simulink model "PurePursuitAlgorithm"  (R2022a)
settings: Solver=ode23t  StartTime=0.0  StopTime=inf  RelTol=1e-3
InitFcn:
  | RPInit
undefined symbols (not defined in the file or in its folder): xRef1, yRef1
libraries: RoboticsPlayground x2
settings Model: Creator=berke  LastModifiedBy=berke
settings DebuggingCC: UnconnectedInputMsg=warning  UnconnectedOutputMsg=warning  UnconnectedLineMsg=warning
settings RTWCC: DLArmComputeVersion=19.05

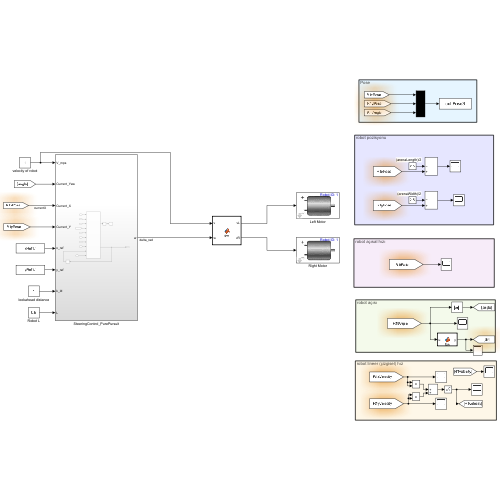
[thumbnail: Simulink's stored preview of the top-level diagram]
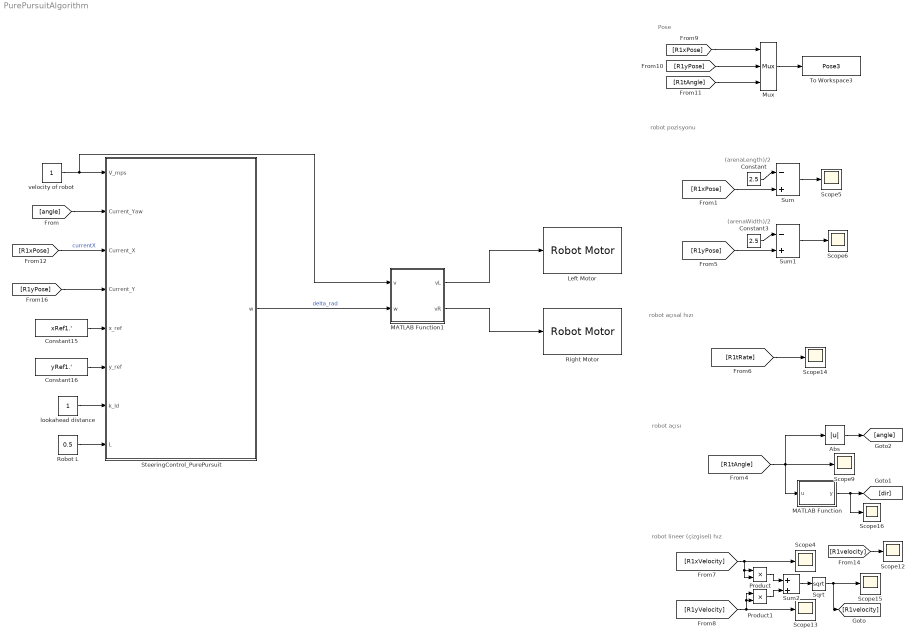
== system PurePursuitAlgorithm ==
  note: robot açısal hızı
  note: robot lineer (çizgisel) hız
  note: robot pozisyonu
  note: robot açısı
  note: (arenaWidth)/2
  note: (arenaLength)/2
  note: Pose
  Abs : Abs  SaturateOnIntegerOverflow=off
  Constant : Constant  Value=2.5
  Constant15 : Constant  Value=xRef1.'  SampleTime=0.01
  Constant16 : Constant  Value=yRef1.'  SampleTime=0.01
  Constant3 : Constant  Value=2.5
  Left Motor : RoboticsPlayground/Basic Sensors and Actuators/Robot Motor  robotId=1  motorChoice=1
      settings: SourceProductName=Robotics Playground
  MATLAB Function : MATLAB Function  TreatAsAtomicUnit=on
  MATLAB Function1 : MATLAB Function  TreatAsAtomicUnit=on
  Mux : Mux  Inputs=3
  Product : Product
  Product1 : Product
  Right Motor : RoboticsPlayground/Basic Sensors and Actuators/Robot Motor  robotId=1  motorChoice=2
      settings: SourceProductName=Robotics Playground
  Robot L : Constant  Value=0.5
  Scope{4..6,9,12..16} (9 alike) : Scope
  Sqrt : Sqrt
  SteeringControl_PurePursuit : Subsystem
  Sum : Sum  Inputs=|-+
  Sum1 : Sum  Inputs=|-+
  Sum2 : Sum  Inputs=|++
  To Workspace3 : ToWorkspace  VariableName=Pose3  SampleTime=-1
  lookahead distance : Constant
  velocity of robot : Constant
  wires:
  lookahead distance/1 -> SteeringControl_PurePursuit/7(k_ld)
  velocity of robot/1 -> MATLAB Function1/1(v), SteeringControl_PurePursuit/1(V_mps)
  [R1velocity] -> Scope12/1
  Constant3/1 -> Sum1/1
  [R1tAngle] -> Mux/3
  [R1xPose] -> Mux/1
  [R1tAngle] -> MATLAB Function/1(u), Abs/1, Scope9/1
  Mux/1 -> To Workspace3/1
  [R1yPose] -> Sum1/2
  Product1/1 -> Sum2/2
  Sum1/1 -> Scope6/1
  Sqrt/1 -> [R1velocity], Scope15/1
  [R1yPose] -> Mux/2
  [R1yVelocity] -> Product1/2, Product1/1, Scope13/1
  [R1xPose] -> Sum/2
  Abs/1 -> [angle]
  MATLAB Function1/2(vR) -> Right Motor/1
  [R1tRate] -> Scope14/1
  Product/1 -> Sum2/1
  [R1xVelocity] -> Product/2, Product/1, Scope4/1
  Sum/1 -> Scope5/1
  Constant/1 -> Sum/1
  MATLAB Function/1(y) -> Scope16/1, [dir]
  Constant16/1 -> SteeringControl_PurePursuit/6(y_ref)
  Constant15/1 -> SteeringControl_PurePursuit/5(x_ref)
  [R1xPose] -> SteeringControl_PurePursuit/3(Current_X)  "currentX"
  [angle] -> SteeringControl_PurePursuit/2(Current_Yaw)
  Sum2/1 -> Sqrt/1
  [R1yPose] -> SteeringControl_PurePursuit/4(Current_Y)
  Robot L/1 -> SteeringControl_PurePursuit/8(L)
  SteeringControl_PurePursuit/1(w) -> MATLAB Function1/2(w)  "delta_rad"
  MATLAB Function1/1(vL) -> Left Motor/1

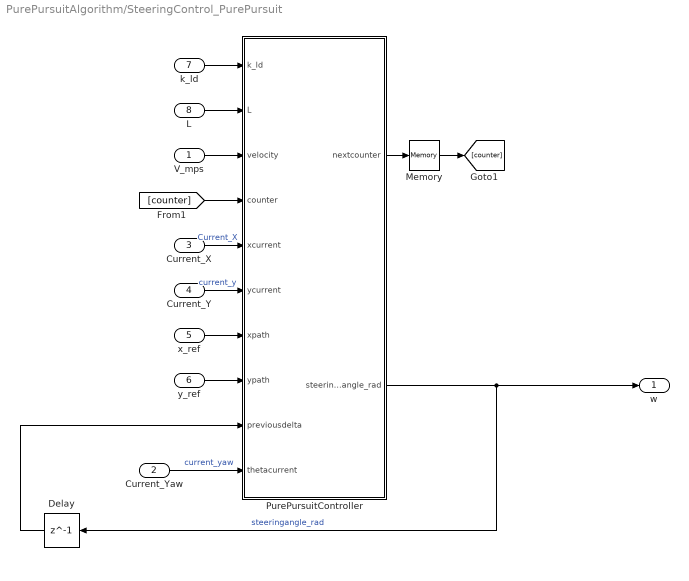
== system PurePursuitAlgorithm/SteeringControl_PurePursuit ==
  V_mps : Inport
  Current_Yaw : Inport  Port=2
  Current_X : Inport  Port=3
  Current_Y : Inport  Port=4
  x_ref : Inport  Port=5
  y_ref : Inport  Port=6
  k_ld : Inport  Port=7
  L : Inport  Port=8
  Delay : Delay  DelayLength=1
  Memory : Memory  InitialCondition=1
  PurePursuitController : MATLAB Function  TreatAsAtomicUnit=on
  w : Outport  VectorParamsAs1DForOutWhenUnconnected=off
  wires:
  Current_Y/1 -> PurePursuitController/6(ycurrent)  "current_y"
  PurePursuitController/2(steering_angle_rad) -> w/1, Delay/1  "steeringangle_rad"
  Current_X/1 -> PurePursuitController/5(xcurrent)  "Current_X"
  [counter] -> PurePursuitController/4(counter)
  PurePursuitController/1(nextcounter) -> Memory/1
  Memory/1 -> [counter]
  V_mps/1 -> PurePursuitController/3(velocity)
  y_ref/1 -> PurePursuitController/8(ypath)
  x_ref/1 -> PurePursuitController/7(xpath)
  Current_Yaw/1 -> PurePursuitController/10(thetacurrent)  "current_yaw"
  k_ld/1 -> PurePursuitController/1(k_ld)
  L/1 -> PurePursuitController/2(L)
  Delay/1 -> PurePursuitController/9(previousdelta)

== matlab function PurePursuitAlgorithm/MATLAB Function1 ==
  data: v input; vL output; w input; vR output
function [vL,vR] = fcn(v,w)
    W = 0.5;
    vL = (2*v - w*W) /2;
    vR = (2*v + w*W) /2;
end

== matlab function PurePursuitAlgorithm/SteeringControl_PurePursuit/PurePursuitController ==
  settings: updateMethod=DISCRETE
  data: k_ld input; L input; velocity input; nextcounter output; counter input; xcurrent input; ycurrent input; xpath input; ypath input; steering_angle_rad output; previousdelta input; thetacurrent input
function [nextcounter,steering_angle_rad] = fcn(k_ld,L, velocity,counter,xcurrent,ycurrent,xpath,ypath,previousdelta,thetacurrent)
delta=previousdelta;
s = size(xpath);

for q=1:10
LookForward=((ypath(counter)-ycurrent)^2+(xpath(counter)-xcurrent)^2)^0.5;
y_path_count=ypath(counter);
x_path_count=xpath(counter);
ld=k_ld*velocity;
if LookForward<ld
    counter=counter+1;
end
    alpha=atan2(ypath(counter)-ycurrent,xpath(counter)-xcurrent)-thetacurrent;
    delta=atan2(2*L*sin(alpha),LookForward);
    
    if counter == s(1)
    counter = 1;
    end
end

nextcounter=counter;


steering_angle_rad =delta;

== matlab function PurePursuitAlgorithm/MATLAB Function ==
  data: u input; y output
function y = fcn(u)
    if u<0
        y=0;
    else
        y=1;
    end

end
